simulink model "IEEE30_case"  (R2024b)
settings: Solver=FixedStepAuto  StartTime=0  StopTime=5  FixedStep=1e-7  RelTol=1e-3
values from neighbouring files (symbols this model uses):
  GFL_DFIG_7_C_bus = 0.08    [IEEE30_case_parameters.m]
  GFL_DFIG_7_D_mutual = 2.500000e+3    (= 2500)    [IEEE30_case_parameters.m]
  GFL_DFIG_7_f0 = 60    [IEEE30_case_parameters.m]
  GFL_DFIG_7_gPLLi = 3200    [IEEE30_case_parameters.m]
  GFL_DFIG_7_gPLLp = 650    [IEEE30_case_parameters.m]
  GFL_DFIG_7_H_WT = 0.4    [IEEE30_case_parameters.m]
  GFL_DFIG_7_Hg = 0.8    [IEEE30_case_parameters.m]
  GFL_DFIG_7_Igq_ref = 0    [IEEE30_case_parameters.m]
  GFL_DFIG_7_Ird_ref = 704.45696    [IEEE30_case_parameters.m]
  GFL_DFIG_7_KI_V = -300000    [IEEE30_case_parameters.m]
  GFL_DFIG_7_KP_V = -1000    [IEEE30_case_parameters.m]
  GFL_DFIG_7_Ksh = 1.254300e+4    (= 12543)    [IEEE30_case_parameters.m]
  GFL_DFIG_7_Lg = 0.000483    [IEEE30_case_parameters.m]
  GFL_DFIG_7_Lm_pu = 4    [IEEE30_case_parameters.m]
  GFL_DFIG_7_N = 100    [IEEE30_case_parameters.m]
  GFL_DFIG_7_p = 2    [IEEE30_case_parameters.m]
  GFL_DFIG_7_Pitch = 0    [IEEE30_case_parameters.m]
  GFL_DFIG_7_R = 44    [IEEE30_case_parameters.m]
  GFL_DFIG_7_Rg = 2.000000e-5    (= 2e-05)    [IEEE30_case_parameters.m]
  GFL_DFIG_7_rho = 1.225    [IEEE30_case_parameters.m]
  GFL_DFIG_7_rPLLi = 4500    [IEEE30_case_parameters.m]
  GFL_DFIG_7_rPLLp = 620    [IEEE30_case_parameters.m]
  GFL_DFIG_7_Rs_pu = 0.011    [IEEE30_case_parameters.m]
  GFL_DFIG_7_Sbase = 2.000000e+6    (= 2000000)    [IEEE30_case_parameters.m]
  GFL_DFIG_7_ugq_ref = 0    [IEEE30_case_parameters.m]
  GFL_DFIG_7_usd_ref = 0    [IEEE30_case_parameters.m]
  GFL_DFIG_7_Vbase = 690    [IEEE30_case_parameters.m]
  GFL_DFIG_7_Vdc_ref = 1200    [IEEE30_case_parameters.m]
  GFL_DFIG_7_wind = 12    [IEEE30_case_parameters.m]
  GFL_DFIG_7_wm_ref = 518.184209    [IEEE30_case_parameters.m]
  SG_D_13_D = 0.01056    [IEEE30_case_parameters.m]
  SG_D_13_EnableSaturation = 0    [IEEE30_case_parameters.m]
  SG_D_13_f0 = 60    [IEEE30_case_parameters.m]
  SG_D_13_H = 7.5    [IEEE30_case_parameters.m]
  SG_D_13_K_A = 20    [IEEE30_case_parameters.m]
  SG_D_13_K_E = 1.000000e+1    (= 10)    [IEEE30_case_parameters.m]
  SG_D_13_K_F = 2.363    [IEEE30_case_parameters.m]
  SG_D_13_K_s = 0.5    [IEEE30_case_parameters.m]
  SG_D_13_R_a = 0.001088    [IEEE30_case_parameters.m]
  SG_D_13_S_A = 1    [IEEE30_case_parameters.m]
  SG_D_13_S_B = 0.103    [IEEE30_case_parameters.m]
  SG_D_13_S_N = 10.659857    [IEEE30_case_parameters.m]
  SG_D_13_SpeedPara = 200    [IEEE30_case_parameters.m]
  SG_D_13_T_0 = 0.370163    [IEEE30_case_parameters.m]
  SG_D_13_T_1 = 0.3    [IEEE30_case_parameters.m]
  SG_D_13_T_2 = 0.05    [IEEE30_case_parameters.m]
  SG_D_13_T_3 = 0.02    [IEEE30_case_parameters.m]
  SG_D_13_T_4 = 0.005    [IEEE30_case_parameters.m]
  SG_D_13_T_A = 0.02    [IEEE30_case_parameters.m]
  SG_D_13_T_dd = 8.000000e+0    (= 8)    [IEEE30_case_parameters.m]
  SG_D_13_T_ddd = 0.04    [IEEE30_case_parameters.m]
  SG_D_13_T_E = 0.314    [IEEE30_case_parameters.m]
  SG_D_13_T_F = 0.35    [IEEE30_case_parameters.m]
  SG_D_13_T_qd = 0.8    [IEEE30_case_parameters.m]
  SG_D_13_T_qdd = 0.02    [IEEE30_case_parameters.m]
  SG_D_13_T_speed = 0.1    [IEEE30_case_parameters.m]
  SG_D_13_T_w = 0.5    [IEEE30_case_parameters.m]
  SG_D_13_V_ref = 1.696619    [IEEE30_case_parameters.m]
  SG_D_13_w_ref = 376.991118    [IEEE30_case_parameters.m]
  SG_D_13_x_d = 1.9    [IEEE30_case_parameters.m]
  SG_D_13_x_dd = 0.302    [IEEE30_case_parameters.m]
  SG_D_13_x_ddd = 0.204    [IEEE30_case_parameters.m]
  SG_D_13_x_l = 0.05    [IEEE30_case_parameters.m]
  SG_D_13_x_q = 1.3    [IEEE30_case_parameters.m]
  SG_D_13_x_qd = 0.5    [IEEE30_case_parameters.m]
  SG_D_13_x_qdd = 0.3    [IEEE30_case_parameters.m]
  SG_D_1_D = 0.01056    [IEEE30_case_parameters.m]
  SG_D_1_EnableSaturation = 0    [IEEE30_case_parameters.m]
  SG_D_1_f0 = 60    [IEEE30_case_parameters.m]
  SG_D_1_H = 7.5    [IEEE30_case_parameters.m]
  SG_D_1_K_A = 20    [IEEE30_case_parameters.m]
  SG_D_1_K_E = 1.000000e+1    (= 10)    [IEEE30_case_parameters.m]
  SG_D_1_K_F = 2.363    [IEEE30_case_parameters.m]
  SG_D_1_K_s = 0.5    [IEEE30_case_parameters.m]
  SG_D_1_R_a = 0.001088    [IEEE30_case_parameters.m]
  SG_D_1_S_A = 1    [IEEE30_case_parameters.m]
  SG_D_1_S_B = 0.103    [IEEE30_case_parameters.m]
  SG_D_1_S_N = 10.659857    [IEEE30_case_parameters.m]
  SG_D_1_SpeedPara = 200    [IEEE30_case_parameters.m]
  SG_D_1_T_0 = 0.259812    [IEEE30_case_parameters.m]
  SG_D_1_T_1 = 0.3    [IEEE30_case_parameters.m]
  SG_D_1_T_2 = 0.05    [IEEE30_case_parameters.m]
  SG_D_1_T_3 = 0.02    [IEEE30_case_parameters.m]
  SG_D_1_T_4 = 0.005    [IEEE30_case_parameters.m]
  SG_D_1_T_A = 0.02    [IEEE30_case_parameters.m]
  SG_D_1_T_dd = 8.000000e+0    (= 8)    [IEEE30_case_parameters.m]
  SG_D_1_T_ddd = 0.04    [IEEE30_case_parameters.m]
  SG_D_1_T_E = 0.314    [IEEE30_case_parameters.m]
  SG_D_1_T_F = 0.35    [IEEE30_case_parameters.m]
  SG_D_1_T_qd = 0.8    [IEEE30_case_parameters.m]
  SG_D_1_T_qdd = 0.02    [IEEE30_case_parameters.m]
  SG_D_1_T_speed = 0.1    [IEEE30_case_parameters.m]
  SG_D_1_T_w = 0.5    [IEEE30_case_parameters.m]
  SG_D_1_V_ref = 1.544107    [IEEE30_case_parameters.m]
  SG_D_1_w_ref = 376.991118    [IEEE30_case_parameters.m]
  SG_D_1_x_d = 1.9    [IEEE30_case_parameters.m]
  SG_D_1_x_dd = 0.302    [IEEE30_case_parameters.m]
  SG_D_1_x_ddd = 0.204    [IEEE30_case_parameters.m]
  SG_D_1_x_l = 0.05    [IEEE30_case_parameters.m]
  SG_D_1_x_q = 1.3    [IEEE30_case_parameters.m]
  SG_D_1_x_qd = 0.5    [IEEE30_case_parameters.m]
  SG_D_1_x_qdd = 0.3    [IEEE30_case_parameters.m]
  SG_D_22_D = 0.01056    [IEEE30_case_parameters.m]
  SG_D_22_EnableSaturation = 0    [IEEE30_case_parameters.m]
  SG_D_22_f0 = 60    [IEEE30_case_parameters.m]
  SG_D_22_H = 7.5    [IEEE30_case_parameters.m]
  SG_D_22_K_A = 20    [IEEE30_case_parameters.m]
  SG_D_22_K_E = 1.000000e+1    (= 10)    [IEEE30_case_parameters.m]
  SG_D_22_K_F = 2.363    [IEEE30_case_parameters.m]
  SG_D_22_K_s = 0.5    [IEEE30_case_parameters.m]
  SG_D_22_R_a = 0.001088    [IEEE30_case_parameters.m]
  SG_D_22_S_A = 1    [IEEE30_case_parameters.m]
  SG_D_22_S_B = 0.103    [IEEE30_case_parameters.m]
  SG_D_22_S_N = 10.659857    [IEEE30_case_parameters.m]
  SG_D_22_SpeedPara = 200    [IEEE30_case_parameters.m]
  SG_D_22_T_0 = 0.216121    [IEEE30_case_parameters.m]
  SG_D_22_T_1 = 0.3    [IEEE30_case_parameters.m]
  SG_D_22_T_2 = 0.05    [IEEE30_case_parameters.m]
  SG_D_22_T_3 = 0.02    [IEEE30_case_parameters.m]
  SG_D_22_T_4 = 0.005    [IEEE30_case_parameters.m]
  ... (+126 more)
(part 16 of 27)

== system IEEE30_case/SG_D_1/d_Px_2_SG_D_1_block ==
  note: d_Px_2_SG_D_1 in IEEE30_case
      | $\frac{\mathrm{Px}_{1,\mathrm{SG},D,1}-T_{2}\,\left(\frac{\mathrm{Px}_{1,\mathrm{SG},D,1}}{T_{w}}-\frac{w_{\mathrm{SG},D,1}-2\,\pi \,f_{0}}{T_{w}}\right)}{T_{1}}-\frac{\mathrm{Px}_{2,\mathrm{SG},D,1}}{T_{1}}$
      | Automatically generated on 2025-11-01 18:30:40 .
  State_Px_2_SG_D_1_7ad78 : Inport
  State_Px_1_SG_D_1_ae78a : Inport  Port=2
  State_Px_1_SG_D_1_3856c : Inport  Port=3
  State_w_SG_D_1_34181 : Inport  Port=4
  Add_14e72 : Sum
  Add_312b6 : Sum
  Add_4af92 : Sum
  Add_c84e5 : Sum
  Constant_-1_0a70e : Constant  Value=-1
  Constant_-1_b2e32 : Constant  Value=-1
  Constant_-2.0_99803 : Constant  Value=-2.0
  Constant_T_1_53d02 : Constant  Value=T_1
  Constant_T_1_b414e : Constant  Value=T_1
  Constant_T_2_fd2a1 : Constant  Value=T_2
  Constant_T_w_8633f : Constant  Value=T_w
  Constant_T_w_a9709 : Constant  Value=T_w
  Constant_f0_f4a44 : Constant  Value=f0
  Constant_pi_968ef : Constant  Value=pi
  Divide_043e7 : Product  Inputs=*/
  Divide_4ff0b : Product  Inputs=*/
  Divide_5a47e : Product  Inputs=*/
  Divide_e1124 : Product  Inputs=*/
  Product_026fd : Product
  Product_1f51f : Product
  Product_38c4f : Product
  Product_a5094 : Product
  Product_e3861 : Product
  Blockout_d_Px_2_SG_D_1_8ee22 : Outport
  wires:
  Constant_-2.0_99803/1 -> Product_1f51f/1
  State_w_SG_D_1_34181/1 -> Add_14e72/2
  Constant_f0_f4a44/1 -> Product_38c4f/2
  Constant_pi_968ef/1 -> Product_1f51f/2
  Add_c84e5/1 -> Product_026fd/2
  Product_38c4f/1 -> Add_14e72/1
  Divide_5a47e/1 -> Add_c84e5/1
  Product_1f51f/1 -> Product_38c4f/1
  Constant_T_w_8633f/1 -> Divide_5a47e/2
  Constant_-1_b2e32/1 -> Product_e3861/1
  State_Px_1_SG_D_1_3856c/1 -> Product_e3861/2
  Divide_e1124/1 -> Add_312b6/1
  Product_e3861/1 -> Divide_5a47e/1
  Add_14e72/1 -> Divide_4ff0b/1
  Constant_T_w_a9709/1 -> Divide_4ff0b/2
  Divide_4ff0b/1 -> Add_c84e5/2
  Constant_T_2_fd2a1/1 -> Product_026fd/1
  Constant_-1_0a70e/1 -> Product_a5094/1
  State_Px_2_SG_D_1_7ad78/1 -> Product_a5094/2
  State_Px_1_SG_D_1_ae78a/1 -> Add_4af92/1
  Product_026fd/1 -> Add_4af92/2
  Add_4af92/1 -> Divide_043e7/1
  Product_a5094/1 -> Divide_e1124/1
  Constant_T_1_b414e/1 -> Divide_e1124/2
  Constant_T_1_53d02/1 -> Divide_043e7/2
  Divide_043e7/1 -> Add_312b6/2
  Add_312b6/1 -> Blockout_d_Px_2_SG_D_1_8ee22/1

== system IEEE30_case/SG_D_1/d_Px_3_SG_D_1_block ==
  note: d_Px_3_SG_D_1 in IEEE30_case
      | $\frac{\mathrm{Px}_{2,\mathrm{SG},D,1}+T_{4}\,\left(\frac{\mathrm{Px}_{1,\mathrm{SG},D,1}-T_{2}\,\left(\frac{\mathrm{Px}_{1,\mathrm{SG},D,1}}{T_{w}}-\frac{w_{\mathrm{SG},D,1}-2\,\pi \,f_{0}}{T_{w}}\right)}{T_{1}}-\frac{\mathrm{Px}_{2,\mathrm{SG},D,1}}{T_{1}}\right)}{T_{3}}-\frac{\mathrm{Px}_{3,\mathrm{SG},D,1}}{T_{3}}$
      | Automatically generated on 2025-11-01 18:30:42 .
  State_Px_3_SG_D_1_caa78 : Inport
  State_Px_2_SG_D_1_d9b49 : Inport  Port=2
  State_Px_2_SG_D_1_ab48e : Inport  Port=3
  State_Px_1_SG_D_1_64472 : Inport  Port=4
  State_Px_1_SG_D_1_665ee : Inport  Port=5
  State_w_SG_D_1_e8e94 : Inport  Port=6
  Add_09c98 : Sum
  Add_369a2 : Sum
  Add_66d7b : Sum
  Add_a0e61 : Sum
  Add_c7021 : Sum
  Add_fc02d : Sum
  Constant_-1_a8f79 : Constant  Value=-1
  Constant_-1_ad1eb : Constant  Value=-1
  Constant_-1_fba85 : Constant  Value=-1
  Constant_-2.0_11787 : Constant  Value=-2.0
  Constant_T_1_05b56 : Constant  Value=T_1
  Constant_T_1_e9ffc : Constant  Value=T_1
  Constant_T_2_5461d : Constant  Value=T_2
  Constant_T_3_767c3 : Constant  Value=T_3
  Constant_T_3_e091a : Constant  Value=T_3
  Constant_T_4_12645 : Constant  Value=T_4
  Constant_T_w_0ee7d : Constant  Value=T_w
  Constant_T_w_88f0f : Constant  Value=T_w
  Constant_f0_a696c : Constant  Value=f0
  Constant_pi_8c04d : Constant  Value=pi
  Divide_5430c : Product  Inputs=*/
  Divide_8ac43 : Product  Inputs=*/
  Divide_bb2bd : Product  Inputs=*/
  Divide_c4060 : Product  Inputs=*/
  Divide_c4299 : Product  Inputs=*/
  Divide_d25e4 : Product  Inputs=*/
  Product_246d8 : Product
  Product_55427 : Product
  Product_581c9 : Product
  Product_5bfea : Product
  Product_96dfd : Product
  Product_c40fa : Product
  Product_cae64 : Product
  Blockout_d_Px_3_SG_D_1_3bf99 : Outport
  wires:
  Constant_T_w_88f0f/1 -> Divide_c4299/2
  Constant_-1_ad1eb/1 -> Product_96dfd/1
  Add_fc02d/1 -> Blockout_d_Px_3_SG_D_1_3bf99/1
  Constant_-2.0_11787/1 -> Product_581c9/1
  State_w_SG_D_1_e8e94/1 -> Add_369a2/2
  Constant_f0_a696c/1 -> Product_cae64/2
  State_Px_1_SG_D_1_665ee/1 -> Product_96dfd/2
  Constant_pi_8c04d/1 -> Product_581c9/2
  Product_cae64/1 -> Add_369a2/1
  Product_581c9/1 -> Product_cae64/1
  Product_96dfd/1 -> Divide_c4299/1
  Divide_bb2bd/1 -> Add_fc02d/1
  Constant_T_3_e091a/1 -> Divide_8ac43/2
  Add_369a2/1 -> Divide_d25e4/1
  Constant_T_w_0ee7d/1 -> Divide_d25e4/2
  Divide_c4299/1 -> Add_a0e61/1
  Divide_d25e4/1 -> Add_a0e61/2
  Constant_-1_fba85/1 -> Product_246d8/1
  Constant_T_2_5461d/1 -> Product_c40fa/1
  Add_a0e61/1 -> Product_c40fa/2
  Constant_-1_a8f79/1 -> Product_5bfea/1
  Divide_8ac43/1 -> Add_fc02d/2
  Constant_T_3_767c3/1 -> Divide_bb2bd/2
  State_Px_2_SG_D_1_ab48e/1 -> Product_5bfea/2
  State_Px_1_SG_D_1_64472/1 -> Add_66d7b/1
  Divide_c4060/1 -> Add_c7021/1
  Product_c40fa/1 -> Add_66d7b/2
  Product_5bfea/1 -> Divide_c4060/1
  Product_246d8/1 -> Divide_bb2bd/1
  Constant_T_1_05b56/1 -> Divide_c4060/2
  Add_66d7b/1 -> Divide_5430c/1
  Constant_T_1_e9ffc/1 -> Divide_5430c/2
  Divide_5430c/1 -> Add_c7021/2
  Constant_T_4_12645/1 -> Product_55427/1
  Add_c7021/1 -> Product_55427/2
  State_Px_3_SG_D_1_caa78/1 -> Product_246d8/2
  State_Px_2_SG_D_1_d9b49/1 -> Add_09c98/1
  Product_55427/1 -> Add_09c98/2
  Add_09c98/1 -> Divide_8ac43/1

== system IEEE30_case/SG_D_1/d_R_f_SG_D_1_block ==
  note: d_R_f_SG_D_1 in IEEE30_case
      | $-\frac{R_{f,\mathrm{SG},D,1}-\frac{E_{\mathrm{fd},\mathrm{SG},D,1}\,K_{F}}{T_{F}}}{T_{F}}$
      | Automatically generated on 2025-11-01 18:30:36 .
  State_E_fd_SG_D_1_7bfd0 : Inport
  State_R_f_SG_D_1_11fa9 : Inport  Port=2
  Constant_K_F_288dd : Constant  Value=K_F
  Constant_T_F_528c7 : Constant  Value=T_F
  Constant_T_F_87a06 : Constant  Value=T_F
  Divide_3eb50 : Product  Inputs=*/
  Divide_9ebff : Product  Inputs=*/
  Product_09a34 : Product
  Subtract_13a9b : Sum  Inputs=+-
  Blockout_d_R_f_SG_D_1_cb206 : Outport
  wires:
  Constant_K_F_288dd/1 -> Product_09a34/2
  Product_09a34/1 -> Divide_3eb50/1
  State_E_fd_SG_D_1_7bfd0/1 -> Product_09a34/1
  State_R_f_SG_D_1_11fa9/1 -> Subtract_13a9b/2
  Constant_T_F_528c7/1 -> Divide_3eb50/2
  Divide_3eb50/1 -> Subtract_13a9b/1
  Divide_9ebff/1 -> Blockout_d_R_f_SG_D_1_cb206/1
  Subtract_13a9b/1 -> Divide_9ebff/1
  Constant_T_F_87a06/1 -> Divide_9ebff/2

== system IEEE30_case/SG_D_1/d_T_m_SG_D_1_block ==
  note: d_T_m_SG_D_1 in IEEE30_case
      | $-\frac{T_{m,\mathrm{SG},D,1}-T_{0}+\frac{\mathrm{SpeedPara}\,\left(w_{\mathrm{SG},D,1}-w_{\mathrm{ref}}\right)}{2\,f_{0}\,\pi }}{T_{\mathrm{speed}}}$
      | Automatically generated on 2025-11-01 18:30:26 .
  State_w_SG_D_1_e56b0 : Inport
  State_T_m_SG_D_1_eb6d8 : Inport  Port=2
  Add_2376c : Sum
  Add_d3f82 : Sum
  Constant_-1_17636 : Constant  Value=-1
  Constant_2.0_24c8d : Constant  Value=2.0
  Constant_SpeedPara_8f4c6 : Constant  Value=SpeedPara
  Constant_T_0_1fdba : Constant  Value=T_0
  Constant_T_speed_8d11c : Constant  Value=T_speed
  Constant_f0_adcf2 : Constant  Value=f0
  Constant_pi_83027 : Constant  Value=pi
  Constant_w_ref_bad2c : Constant  Value=w_ref
  Divide_03ba9 : Product  Inputs=*/
  Divide_931b1 : Product  Inputs=*/
  Product_038ba : Product
  Product_39944 : Product
  Product_c8531 : Product
  Product_eec2d : Product
  Subtract_6dd9b : Sum  Inputs=+-
  Blockout_d_T_m_SG_D_1_12514 : Outport
  wires:
  Constant_-1_17636/1 -> Product_39944/1
  Constant_w_ref_bad2c/1 -> Add_d3f82/2
  State_w_SG_D_1_e56b0/1 -> Product_39944/2
  Add_2376c/1 -> Subtract_6dd9b/1
  Add_d3f82/1 -> Product_038ba/2
  Product_39944/1 -> Add_d3f82/1
  Constant_2.0_24c8d/1 -> Product_eec2d/1
  Constant_pi_83027/1 -> Product_eec2d/2
  Constant_SpeedPara_8f4c6/1 -> Product_038ba/1
  Product_eec2d/1 -> Product_c8531/1
  Constant_f0_adcf2/1 -> Product_c8531/2
  Constant_T_speed_8d11c/1 -> Divide_931b1/2
  Product_038ba/1 -> Divide_03ba9/1
  Product_c8531/1 -> Divide_03ba9/2
  Divide_03ba9/1 -> Add_2376c/1
  Constant_T_0_1fdba/1 -> Add_2376c/2
  State_T_m_SG_D_1_eb6d8/1 -> Subtract_6dd9b/2
  Subtract_6dd9b/1 -> Divide_931b1/1
  Divide_931b1/1 -> Blockout_d_T_m_SG_D_1_12514/1

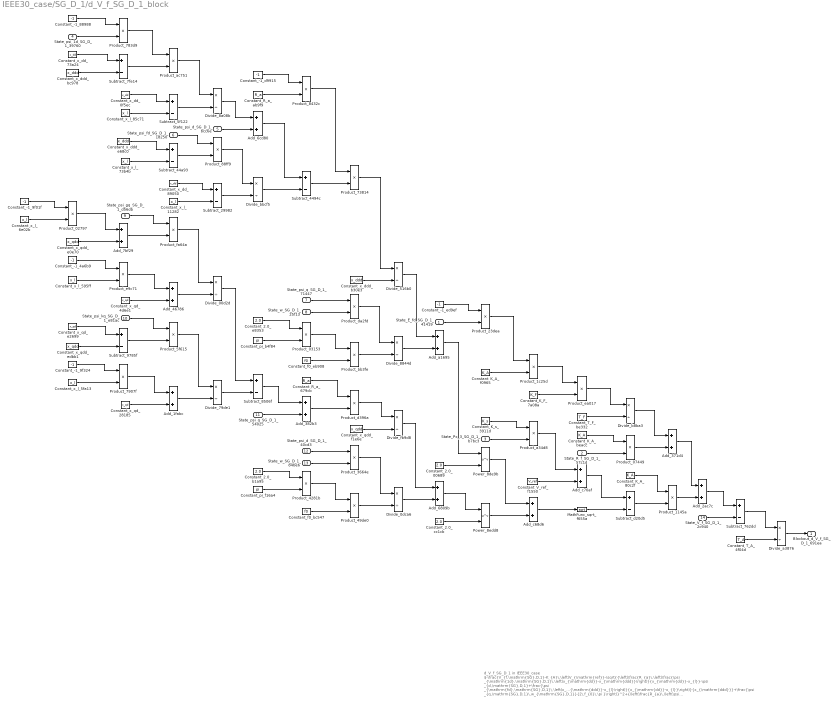
== system IEEE30_case/SG_D_1/d_V_f_SG_D_1_block ==
  note: d_V_f_SG_D_1 in IEEE30_case
      | $-\frac{V_{f,\mathrm{SG},D,1}-K_{A}\,\left(V_{\mathrm{ref}}-\sqrt{{\left(\frac{R_{a}\,\left(\frac{\psi _{\mathrm{1d},\mathrm{SG},D,1}\,\left(x_{\mathrm{dd}}-x_{\mathrm{ddd}}\right)}{x_{\mathrm{dd}}-x_{l}}-\psi _{d,\mathrm{SG},D,1}+\frac{\psi _{\mathrm{fd},\mathrm{SG},D,1}\,\left(x_{\mathrm{ddd}}-x_{l}\right)}{x_{\mathrm{dd}}-x_{l}}\right)}{x_{\mathrm{ddd}}}+\frac{\psi _{q,\mathrm{SG},D,1}\,w_{\mathrm{SG},D,1}}{2\,f_{0}\,\pi }\right)}^2+{\left(\frac{R_{a}\,\left(\psi _{q,\mathrm{SG},D,1}+\frac{\psi _{\mathrm{gq},\mathrm{SG},D,1}\,\left(x_{l}-x_{\mathrm{qdd}}\right)}{x_{l}-x_{\mathrm{qd}}}+\frac{\psi _{\mathrm{kq},\mathrm{SG},D,1}\,\left(x_{\mathrm{qd}}-x_{\mathrm{qdd}}\right)}{x_{l}-x_{\mathrm{qd}}}\right)}{x_{\mathrm{qdd}}}+\frac{\psi _{d,\mathrm{SG},D,1}\,w_{\mathrm{SG},D,1}}{2\,f_{0}\,\pi }\right)}^2}+K_{s}\,\mathrm{Px}_{3,\mathrm{SG},D,1}\right)-K_{A}\,R_{f,\mathrm{SG},D,1}+\frac{E_{\mathrm{fd},\mathrm{SG},D,1}\,K_{A}\,K_{F}}{T_{F}}}{T_{A}}$
      | Automatically generated on 2025-11-01 18:30:34 .
  State_E_fd_SG_D_1_41419 : Inport
  State_R_f_SG_D_1_57c1d : Inport  Port=2
  State_Px_3_SG_D_1_b7bc3 : Inport  Port=3
  State_psi_1d_SG_D_1_39760 : Inport  Port=4
  State_psi_d_SG_D_1_bcc6e : Inport  Port=5
  State_psi_fd_SG_D_1_18250 : Inport  Port=6
  State_psi_q_SG_D_1_71447 : Inport  Port=7
  State_w_SG_D_1_25f13 : Inport  Port=8
  State_psi_gq_SG_D_1_d56db : Inport  Port=9
  State_psi_kq_SG_D_1_e81ac : Inport  Port=10
  State_psi_q_SG_D_1_54025 : Inport  Port=11
  State_psi_d_SG_D_1_40cd3 : Inport  Port=12
  State_w_SG_D_1_84be6 : Inport  Port=13
  State_V_f_SG_D_1_2c940 : Inport  Port=14
  Add_1fabc : Sum
  Add_2ac7c : Sum
  Add_371d4 : Sum
  Add_382b3 : Sum
  Add_46786 : Sum
  Add_6809b : Sum
  Add_6cd80 : Sum
  Add_7bf29 : Sum
  Add_a1695 : Sum
  Add_c68d6 : Sum
  Add_c70af : Sum
  Constant_-1_4a6b9 : Constant  Value=-1
  Constant_-1_88988 : Constant  Value=-1
  Constant_-1_9f01f : Constant  Value=-1
  Constant_-1_9f324 : Constant  Value=-1
  Constant_-1_d9915 : Constant  Value=-1
  Constant_-1_ed9ef : Constant  Value=-1
  Constant_2.0_00689 : Constant  Value=2.0
  Constant_2.0_b1a95 : Constant  Value=2.0
  Constant_2.0_cc1cb : Constant  Value=2.0
  Constant_2.0_e8353 : Constant  Value=2.0
  Constant_K_A_80c2f : Constant  Value=K_A
  Constant_K_A_beacc : Constant  Value=K_A
  Constant_K_A_f0965 : Constant  Value=K_A
  Constant_K_F_7a08a : Constant  Value=K_F
  Constant_K_s_3911d : Constant  Value=K_s
  Constant_R_a_679cb : Constant  Value=R_a
  Constant_R_a_ab9f9 : Constant  Value=R_a
  Constant_T_A_4f04d : Constant  Value=T_A
  Constant_T_F_be332 : Constant  Value=T_F
  Constant_V_ref_f1550 : Constant  Value=V_ref
  Constant_f0_bc547 : Constant  Value=f0
  Constant_f0_eb908 : Constant  Value=f0
  Constant_pi_b4f84 : Constant  Value=pi
  Constant_pi_f16a4 : Constant  Value=pi
  Constant_x_dd_0f5ec : Constant  Value=x_dd
  Constant_x_dd_73a24 : Constant  Value=x_dd
  Constant_x_dd_89050 : Constant  Value=x_dd
  Constant_x_ddd_b30e3 : Constant  Value=x_ddd
  Constant_x_ddd_bc978 : Constant  Value=x_ddd
  Constant_x_ddd_e68c0 : Constant  Value=x_ddd
  Constant_x_l_11282 : Constant  Value=x_l
  Constant_x_l_595ff : Constant  Value=x_l
  Constant_x_l_5fa13 : Constant  Value=x_l
  Constant_x_l_6e02b : Constant  Value=x_l
  Constant_x_l_73b4b : Constant  Value=x_l
  Constant_x_l_85c71 : Constant  Value=x_l
  Constant_x_qd_28185 : Constant  Value=x_qd
  Constant_x_qd_4d6e1 : Constant  Value=x_qd
  Constant_x_qd_e2699 : Constant  Value=x_qd
  Constant_x_qdd_e0e70 : Constant  Value=x_qdd
  Constant_x_qdd_edbb1 : Constant  Value=x_qdd
  Constant_x_qdd_f1e6e : Constant  Value=x_qdd
  Divide_00d2d : Product  Inputs=*/
  Divide_0dca6 : Product  Inputs=*/
  Divide_516b0 : Product  Inputs=*/
  Divide_79de1 : Product  Inputs=*/
  Divide_8844d : Product  Inputs=*/
  Divide_8a08b : Product  Inputs=*/
  Divide_a3876 : Product  Inputs=*/
  Divide_b8ba3 : Product  Inputs=*/
  Divide_bbcf5 : Product  Inputs=*/
  Divide_fb9d8 : Product  Inputs=*/
  MathFunc_sqrt_f655a : Sqrt
  Power_8de9b : Math  Operator=pow
  Power_8edd8 : Math  Operator=pow
  Product_02797 : Product
  Product_03153 : Product
  Product_07449 : Product
  Product_1145a : Product
  Product_1c25d : Product
  Product_23dea : Product
  Product_3664e : Product
  Product_4281b : Product
  Product_49de0 : Product
  Product_5f615 : Product
  Product_73814 : Product
  Product_783d9 : Product
  Product_7907f : Product
  Product_8432c : Product
  Product_88ff9 : Product
  Product_a34d8 : Product
  Product_ac751 : Product
  Product_bb3fe : Product
  Product_d396a : Product
  Product_da2fd : Product
  Product_e9c71 : Product
  Product_ea017 : Product
  Product_fa64a : Product
  Subtract_29982 : Sum  Inputs=+-
  Subtract_4494c : Sum  Inputs=+-
  Subtract_44a93 : Sum  Inputs=+-
  Subtract_5f122 : Sum  Inputs=+-
  Subtract_762dd : Sum  Inputs=+-
  Subtract_7fe14 : Sum  Inputs=+-
  Subtract_8506f : Sum  Inputs=+-
  Subtract_9785f : Sum  Inputs=+-
  Subtract_d20d5 : Sum  Inputs=+-
  Blockout_d_V_f_SG_D_1_691ea : Outport
  wires:
  Constant_-1_9f324/1 -> Product_7907f/1
  Constant_-1_9f01f/1 -> Product_02797/1
  State_psi_d_SG_D_1_40cd3/1 -> Product_3664e/1
  Constant_x_qd_28185/1 -> Add_1fabc/2
  Constant_x_qdd_e0e70/1 -> Add_7bf29/2
  State_w_SG_D_1_84be6/1 -> Product_3664e/2
  Constant_x_l_6e02b/1 -> Product_02797/2
  Subtract_4494c/1 -> Product_73814/2
  Constant_x_l_5fa13/1 -> Product_7907f/2
  Constant_x_dd_73a24/1 -> Subtract_7fe14/1
  Constant_R_a_ab9f9/1 -> Product_8432c/2
  Constant_-1_88988/1 -> Product_783d9/1
  Divide_bbcf5/1 -> Subtract_4494c/2
  Constant_x_ddd_bc978/1 -> Subtract_7fe14/2
  Add_1fabc/1 -> Divide_79de1/2
  State_psi_1d_SG_D_1_39760/1 -> Product_783d9/2
  Add_46786/1 -> Divide_00d2d/2
  Subtract_9785f/1 -> Product_5f615/2
  Product_ea017/1 -> Divide_b8ba3/1
  Product_03153/1 -> Product_bb3fe/1
  Product_02797/1 -> Add_7bf29/1
  Constant_-1_4a6b9/1 -> Product_e9c71/1
  Constant_x_l_595ff/1 -> Product_e9c71/2
  Add_6cd80/1 -> Subtract_4494c/1
  Constant_2.0_b1a95/1 -> Product_4281b/1
  Constant_x_qd_e2699/1 -> Subtract_9785f/1
  Product_783d9/1 -> Product_ac751/1
  Constant_pi_f16a4/1 -> Product_4281b/2
  Constant_x_qdd_edbb1/1 -> Subtract_9785f/2
  Subtract_7fe14/1 -> Product_ac751/2
  State_psi_q_SG_D_1_54025/1 -> Add_382b3/2
  Constant_x_dd_0f5ec/1 -> Subtract_5f122/1
  Constant_x_l_85c71/1 -> Subtract_5f122/2
  Constant_x_ddd_e68c0/1 -> Subtract_44a93/1
  Constant_x_l_73b4b/1 -> Subtract_44a93/2
  State_psi_gq_SG_D_1_d56db/1 -> Product_fa64a/1
  Add_7bf29/1 -> Product_fa64a/2
  Product_e9c71/1 -> Add_46786/1
  Constant_x_qd_4d6e1/1 -> Add_46786/2
  Divide_8a08b/1 -> Add_6cd80/1
  Subtract_5f122/1 -> Divide_8a08b/2
  State_psi_kq_SG_D_1_e81ac/1 -> Product_5f615/1
  Divide_a3876/1 -> Blockout_d_V_f_SG_D_1_691ea/1
  Product_7907f/1 -> Add_1fabc/1
  Product_ac751/1 -> Divide_8a08b/1
  State_psi_fd_SG_D_1_18250/1 -> Product_88ff9/1
  State_w_SG_D_1_25f13/1 -> Product_da2fd/2
  Subtract_44a93/1 -> Product_88ff9/2
  Constant_x_dd_89050/1 -> Subtract_29982/1
  Constant_x_l_11282/1 -> Subtract_29982/2
  Product_fa64a/1 -> Divide_00d2d/1
  Product_8432c/1 -> Product_73814/1
  Product_5f615/1 -> Divide_79de1/1
  State_psi_d_SG_D_1_bcc6e/1 -> Add_6cd80/2
  Product_88ff9/1 -> Divide_bbcf5/1
  Subtract_29982/1 -> Divide_bbcf5/2
  Divide_00d2d/1 -> Subtract_8506f/1
  Divide_79de1/1 -> Subtract_8506f/2
  Constant_-1_d9915/1 -> Product_8432c/1
  Constant_2.0_e8353/1 -> Product_03153/1
  Constant_pi_b4f84/1 -> Product_03153/2
  Subtract_8506f/1 -> Add_382b3/1
  State_psi_q_SG_D_1_71447/1 -> Product_da2fd/1
  Constant_f0_eb908/1 -> Product_bb3fe/2
  Constant_R_a_679cb/1 -> Product_d396a/1
  Add_382b3/1 -> Product_d396a/2
  Product_4281b/1 -> Product_49de0/1
  Power_8de9b/1 -> Add_c68d6/1
  Constant_f0_bc547/1 -> Product_49de0/2
  Product_73814/1 -> Divide_516b0/1
  Constant_x_ddd_b30e3/1 -> Divide_516b0/2
  Product_da2fd/1 -> Divide_8844d/1
  Product_bb3fe/1 -> Divide_8844d/2
  Product_d396a/1 -> Divide_fb9d8/1
  Constant_x_qdd_f1e6e/1 -> Divide_fb9d8/2
  Product_3664e/1 -> Divide_0dca6/1
  Product_49de0/1 -> Divide_0dca6/2
  Divide_516b0/1 -> Add_a1695/1
  Divide_8844d/1 -> Add_a1695/2
  Divide_fb9d8/1 -> Add_6809b/1
  Divide_0dca6/1 -> Add_6809b/2
  Constant_-1_ed9ef/1 -> Product_23dea/1
  State_E_fd_SG_D_1_41419/1 -> Product_23dea/2
  Add_a1695/1 -> Power_8de9b/1
  Constant_2.0_00689/1 -> Power_8de9b/2
  Add_6809b/1 -> Power_8edd8/1
  Constant_2.0_cc1cb/1 -> Power_8edd8/2
  Product_23dea/1 -> Product_1c25d/1
  Constant_K_A_f0965/1 -> Product_1c25d/2
  Constant_K_s_3911d/1 -> Product_a34d8/1
  State_Px_3_SG_D_1_b7bc3/1 -> Product_a34d8/2
  Power_8edd8/1 -> Add_c68d6/2
  Divide_b8ba3/1 -> Add_371d4/1
  Product_1c25d/1 -> Product_ea017/1
  Constant_K_F_7a08a/1 -> Product_ea017/2
  Product_a34d8/1 -> Add_c70af/1
  Constant_V_ref_f1550/1 -> Add_c70af/2
  Add_c68d6/1 -> MathFunc_sqrt_f655a/1
  Constant_T_F_be332/1 -> Divide_b8ba3/2
  Constant_K_A_beacc/1 -> Product_07449/1
  State_R_f_SG_D_1_57c1d/1 -> Product_07449/2
  Add_c70af/1 -> Subtract_d20d5/1
  MathFunc_sqrt_f655a/1 -> Subtract_d20d5/2
  Constant_T_A_4f04d/1 -> Divide_a3876/2
  Product_07449/1 -> Add_371d4/2
  Constant_K_A_80c2f/1 -> Product_1145a/1
  Subtract_d20d5/1 -> Product_1145a/2
  Add_371d4/1 -> Add_2ac7c/1
  Product_1145a/1 -> Add_2ac7c/2
  Add_2ac7c/1 -> Subtract_762dd/1
  State_V_f_SG_D_1_2c940/1 -> Subtract_762dd/2
  Subtract_762dd/1 -> Divide_a3876/1

== system IEEE30_case/SG_D_1/d_psi_1d_SG_D_1_block ==
  note: d_psi_1d_SG_D_1 in IEEE30_case
      | $-\frac{\psi _{\mathrm{1d},\mathrm{SG},D,1}-\psi _{\mathrm{fd},\mathrm{SG},D,1}+\frac{\left(x_{\mathrm{dd}}-x_{l}\right)\,\left(\frac{\psi _{\mathrm{1d},\mathrm{SG},D,1}\,\left(x_{\mathrm{dd}}-x_{\mathrm{ddd}}\right)}{x_{\mathrm{dd}}-x_{l}}-\psi _{d,\mathrm{SG},D,1}+\frac{\psi _{\mathrm{fd},\mathrm{SG},D,1}\,\left(x_{\mathrm{ddd}}-x_{l}\right)}{x_{\mathrm{dd}}-x_{l}}\right)}{x_{\mathrm{ddd}}}}{T_{\mathrm{ddd}}}$
      | Automatically generated on 2025-11-01 18:30:08 .
  State_psi_1d_SG_D_1_acde6 : Inport
  State_psi_fd_SG_D_1_697dc : Inport  Port=2
  State_psi_1d_SG_D_1_d153a : Inport  Port=3
  State_psi_d_SG_D_1_ee12b : Inport  Port=4
  State_psi_fd_SG_D_1_a7ee9 : Inport  Port=5
  Add_5282d : Sum
  Add_52e71 : Sum
  Add_8db4e : Sum
  Constant_-1_12fb9 : Constant  Value=-1
  Constant_-1_da2b3 : Constant  Value=-1
  Constant_T_ddd_a3ac7 : Constant  Value=T_ddd
  Constant_x_dd_811ab : Constant  Value=x_dd
  Constant_x_dd_9202a : Constant  Value=x_dd
  Constant_x_dd_93c5d : Constant  Value=x_dd
  Constant_x_dd_b2d25 : Constant  Value=x_dd
  Constant_x_ddd_22811 : Constant  Value=x_ddd
  Constant_x_ddd_71fa5 : Constant  Value=x_ddd
  Constant_x_ddd_90b96 : Constant  Value=x_ddd
  Constant_x_l_1248a : Constant  Value=x_l
  Constant_x_l_4abbc : Constant  Value=x_l
  Constant_x_l_52946 : Constant  Value=x_l
  Constant_x_l_85f89 : Constant  Value=x_l
  Divide_024ae : Product  Inputs=*/
  Divide_23a68 : Product  Inputs=*/
  Divide_6eb96 : Product  Inputs=*/
  Divide_acb20 : Product  Inputs=*/
  Product_30929 : Product
  Product_739fc : Product
  Product_9bbd6 : Product
  Product_d4260 : Product
  Product_d919b : Product
  Subtract_21dd2 : Sum  Inputs=+-
  Subtract_3d153 : Sum  Inputs=+-
  Subtract_7c245 : Sum  Inputs=+-
  Subtract_8b3b8 : Sum  Inputs=+-
  Subtract_9628b : Sum  Inputs=+-
  Subtract_e1559 : Sum  Inputs=+-
  Blockout_d_psi_1d_SG_D_1_c059e : Outport
  wires:
  Product_d919b/1 -> Product_9bbd6/1
  Constant_-1_12fb9/1 -> Product_d919b/1
  Subtract_7c245/1 -> Product_9bbd6/2
  State_psi_1d_SG_D_1_d153a/1 -> Product_d919b/2
  Subtract_9628b/1 -> Product_30929/1
  State_psi_d_SG_D_1_ee12b/1 -> Add_52e71/2
  Constant_x_dd_b2d25/1 -> Subtract_8b3b8/1
  Constant_x_l_85f89/1 -> Subtract_9628b/2
  Constant_x_dd_811ab/1 -> Subtract_7c245/1
  Subtract_3d153/1 -> Product_d4260/2
  Constant_x_l_1248a/1 -> Subtract_8b3b8/2
  Divide_acb20/1 -> Subtract_21dd2/2
  Constant_x_ddd_90b96/1 -> Subtract_7c245/2
  Constant_x_ddd_71fa5/1 -> Subtract_3d153/1
  Constant_x_l_4abbc/1 -> Subtract_3d153/2
  Add_8db4e/1 -> Add_5282d/1
  Product_9bbd6/1 -> Divide_6eb96/1
  Divide_23a68/1 -> Add_5282d/2
  Subtract_8b3b8/1 -> Divide_6eb96/2
  State_psi_fd_SG_D_1_a7ee9/1 -> Product_d4260/1
  Constant_x_dd_9202a/1 -> Subtract_e1559/1
  Constant_x_l_52946/1 -> Subtract_e1559/2
  Constant_x_ddd_22811/1 -> Divide_23a68/2
  Subtract_21dd2/1 -> Product_30929/2
  Divide_6eb96/1 -> Add_52e71/1
  Product_d4260/1 -> Divide_acb20/1
  Subtract_e1559/1 -> Divide_acb20/2
  Product_30929/1 -> Divide_23a68/1
  Constant_x_dd_93c5d/1 -> Subtract_9628b/1
  Add_52e71/1 -> Subtract_21dd2/1
  Constant_-1_da2b3/1 -> Product_739fc/1
  State_psi_1d_SG_D_1_acde6/1 -> Product_739fc/2
  Product_739fc/1 -> Add_8db4e/1
  State_psi_fd_SG_D_1_697dc/1 -> Add_8db4e/2
  Add_5282d/1 -> Divide_024ae/1
  Constant_T_ddd_a3ac7/1 -> Divide_024ae/2
  Divide_024ae/1 -> Blockout_d_psi_1d_SG_D_1_c059e/1

== system IEEE30_case/SG_D_1/d_psi_d_SG_D_1_block ==
  note: d_psi_d_SG_D_1 in IEEE30_case
      | $2\,\pi \,f_{0}\,\left(v_{d,\mathrm{SG},D,1}\,\sin\left(\theta _{\mathrm{SG},D,1}\right)-v_{q,\mathrm{SG},D,1}\,\cos\left(\theta _{\mathrm{SG},D,1}\right)+\frac{R_{a}\,\left(\frac{\psi _{\mathrm{1d},\mathrm{SG},D,1}\,\left(x_{\mathrm{dd}}-x_{\mathrm{ddd}}\right)}{x_{\mathrm{dd}}-x_{l}}-\psi _{d,\mathrm{SG},D,1}+\frac{\psi _{\mathrm{fd},\mathrm{SG},D,1}\,\left(x_{\mathrm{ddd}}-x_{l}\right)}{x_{\mathrm{dd}}-x_{l}}\right)}{x_{\mathrm{ddd}}}+\frac{\psi _{q,\mathrm{SG},D,1}\,w_{\mathrm{SG},D,1}}{2\,f_{0}\,\pi }\right)$
      | Automatically generated on 2025-11-01 18:29:41 .
  State_psi_1d_SG_D_1_5396e : Inport
  State_psi_d_SG_D_1_d85a6 : Inport  Port=2
  State_psi_fd_SG_D_1_f658e : Inport  Port=3
  Input_v_d_SG_D_1_95be5 : Inport  Port=4
  State_theta_SG_D_1_3e828 : Inport  Port=5
  Input_v_q_SG_D_1_f5767 : Inport  Port=6
  State_theta_SG_D_1_93c49 : Inport  Port=7
  State_psi_q_SG_D_1_efd17 : Inport  Port=8
  State_w_SG_D_1_d2cfd : Inport  Port=9
  Add_b2cc0 : Sum
  Add_ec660 : Sum
  Constant_-1_38384 : Constant  Value=-1
  Constant_-2.0_0cf5a : Constant  Value=-2.0
  Constant_2.0_3349a : Constant  Value=2.0
  Constant_R_a_b96de : Constant  Value=R_a
  Constant_f0_4de23 : Constant  Value=f0
  Constant_f0_53b7b : Constant  Value=f0
  Constant_pi_47aad : Constant  Value=pi
  Constant_pi_fd6f4 : Constant  Value=pi
  Constant_x_dd_45d12 : Constant  Value=x_dd
  Constant_x_dd_8310c : Constant  Value=x_dd
  Constant_x_dd_a5eb8 : Constant  Value=x_dd
  Constant_x_ddd_6a29b : Constant  Value=x_ddd
  Constant_x_ddd_832ed : Constant  Value=x_ddd
  Constant_x_ddd_e6836 : Constant  Value=x_ddd
  Constant_x_l_25dcd : Constant  Value=x_l
  Constant_x_l_5e9da : Constant  Value=x_l
  Constant_x_l_ffce5 : Constant  Value=x_l
  Divide_128e2 : Product  Inputs=*/
  Divide_489db : Product  Inputs=*/
  Divide_a41a9 : Product  Inputs=*/
  Divide_c2f47 : Product  Inputs=*/
  MathFunc_cos_86319 : Trigonometry  Operator=cos
  MathFunc_sin_afe2a : Trigonometry
  Product_21064 : Product
  Product_3c407 : Product
  Product_7a831 : Product
  Product_7ef06 : Product
  Product_8cdae : Product
  Product_8d80b : Product
  Product_932e8 : Product
  Product_ba84c : Product
  Product_c21e8 : Product
  Product_cb69a : Product
  Product_e5f81 : Product
  Product_f731f : Product
  Subtract_4b3ee : Sum  Inputs=+-
  Subtract_5a4a0 : Sum  Inputs=+-
  Subtract_6b146 : Sum  Inputs=+-
  Subtract_84717 : Sum  Inputs=+-
  Subtract_a6f20 : Sum  Inputs=+-
  Subtract_aa1cc : Sum  Inputs=+-
  Subtract_dffd2 : Sum  Inputs=+-
  Blockout_d_psi_d_SG_D_1_2866c : Outport
  wires:
  Add_b2cc0/1 -> Subtract_dffd2/1
  Product_7ef06/1 -> Divide_c2f47/1
  Subtract_aa1cc/1 -> Product_7ef06/2
  Divide_c2f47/1 -> Add_b2cc0/1
  Product_3c407/1 -> Product_7ef06/1
  Constant_x_ddd_e6836/1 -> Subtract_aa1cc/2
  Constant_x_dd_45d12/1 -> Subtract_aa1cc/1
  State_psi_1d_SG_D_1_5396e/1 -> Product_3c407/2
  Constant_-1_38384/1 -> Product_3c407/1
  Product_21064/1 -> Divide_128e2/1
  Constant_x_l_ffce5/1 -> Subtract_84717/2
  State_psi_d_SG_D_1_d85a6/1 -> Add_b2cc0/2
  Constant_x_dd_a5eb8/1 -> Subtract_84717/1
  Constant_x_ddd_832ed/1 -> Subtract_a6f20/1
  Constant_x_l_25dcd/1 -> Subtract_a6f20/2
  Subtract_84717/1 -> Divide_c2f47/2
  State_psi_fd_SG_D_1_f658e/1 -> Product_21064/1
  Constant_x_ddd_6a29b/1 -> Divide_489db/2
  Subtract_a6f20/1 -> Product_21064/2
  Product_932e8/1 -> Subtract_5a4a0/2
  Constant_x_dd_8310c/1 -> Subtract_6b146/1
  Constant_x_l_5e9da/1 -> Subtract_6b146/2
  Subtract_6b146/1 -> Divide_128e2/2
  Divide_128e2/1 -> Subtract_dffd2/2
  Constant_R_a_b96de/1 -> Product_e5f81/1
  Subtract_dffd2/1 -> Product_e5f81/2
  MathFunc_cos_86319/1 -> Product_ba84c/2
  State_theta_SG_D_1_3e828/1 -> MathFunc_sin_afe2a/1
  Divide_489db/1 -> Subtract_5a4a0/1
  Product_e5f81/1 -> Divide_489db/1
  MathFunc_sin_afe2a/1 -> Product_932e8/2
  Input_v_d_SG_D_1_95be5/1 -> Product_932e8/1
  Product_8cdae/1 -> Blockout_d_psi_d_SG_D_1_2866c/1
  Product_f731f/1 -> Product_8cdae/1
  Product_7a831/1 -> Product_f731f/1
  State_theta_SG_D_1_93c49/1 -> MathFunc_cos_86319/1
  Constant_2.0_3349a/1 -> Product_8d80b/1
  Constant_pi_47aad/1 -> Product_8d80b/2
  Input_v_q_SG_D_1_f5767/1 -> Product_ba84c/1
  Constant_f0_53b7b/1 -> Product_f731f/2
  State_psi_q_SG_D_1_efd17/1 -> Product_cb69a/1
  State_w_SG_D_1_d2cfd/1 -> Product_cb69a/2
  Product_8d80b/1 -> Product_c21e8/1
  Constant_pi_fd6f4/1 -> Product_7a831/2
  Constant_f0_4de23/1 -> Product_c21e8/2
  Constant_-2.0_0cf5a/1 -> Product_7a831/1
  Add_ec660/1 -> Subtract_4b3ee/1
  Subtract_5a4a0/1 -> Add_ec660/1
  Product_ba84c/1 -> Add_ec660/2
  Product_cb69a/1 -> Divide_a41a9/1
  Product_c21e8/1 -> Divide_a41a9/2
  Divide_a41a9/1 -> Subtract_4b3ee/2
  Subtract_4b3ee/1 -> Product_8cdae/2

== system IEEE30_case/SG_D_1/d_psi_fd_SG_D_1_block ==
  note: d_psi_fd_SG_D_1 in IEEE30_case
      | $-\frac{\psi _{\mathrm{fd},\mathrm{SG},D,1}-E_{\mathrm{fd},\mathrm{SG},D,1}+\left(x_{d}-x_{\mathrm{dd}}\right)\,\left(\frac{\frac{\psi _{\mathrm{1d},\mathrm{SG},D,1}\,\left(x_{\mathrm{dd}}-x_{\mathrm{ddd}}\right)}{x_{\mathrm{dd}}-x_{l}}-\psi _{d,\mathrm{SG},D,1}+\frac{\psi _{\mathrm{fd},\mathrm{SG},D,1}\,\left(x_{\mathrm{ddd}}-x_{l}\right)}{x_{\mathrm{dd}}-x_{l}}}{x_{\mathrm{ddd}}}-\frac{\left(x_{\mathrm{dd}}-x_{\mathrm{ddd}}\right)\,\left(\psi _{\mathrm{1d},\mathrm{SG},D,1}-\psi _{\mathrm{fd},\mathrm{SG},D,1}+\frac{\left(x_{\mathrm{dd}}-x_{l}\right)\,\left(\frac{\psi _{\mathrm{1d},\mathrm{SG},D,1}\,\left(x_{\mathrm{dd}}-x_{\mathrm{ddd}}\right)}{x_{\mathrm{dd}}-x_{l}}-\psi _{d,\mathrm{SG},D,1}+\frac{\psi _{\mathrm{fd},\mathrm{SG},D,1}\,\left(x_{\mathrm{ddd}}-x_{l}\right)}{x_{\mathrm{dd}}-x_{l}}\right)}{x_{\mathrm{ddd}}}\right)}{{\left(x_{\mathrm{dd}}-x_{l}\right)}^2}\right)}{T_{\mathrm{dd}}}$
      | Automatically generated on 2025-11-01 18:30:06 .
  State_E_fd_SG_D_1_d5aee : Inport
  State_psi_fd_SG_D_1_c7574 : Inport  Port=2
  State_psi_1d_SG_D_1_1742e : Inport  Port=3
  State_psi_fd_SG_D_1_fe3bf : Inport  Port=4
  State_psi_1d_SG_D_1_b3018 : Inport  Port=5
  State_psi_d_SG_D_1_a13b4 : Inport  Port=6
  State_psi_fd_SG_D_1_1eed0 : Inport  Port=7
  State_psi_1d_SG_D_1_10652 : Inport  Port=8
  State_psi_d_SG_D_1_482bf : Inport  Port=9
  State_psi_fd_SG_D_1_e31c3 : Inport  Port=10
  Add_1720d : Sum
  Add_bb906 : Sum
  Constant_-1_1333f : Constant  Value=-1
  Constant_-1_82476 : Constant  Value=-1
  Constant_-1_82d8b : Constant  Value=-1
  Constant_2.0_a0827 : Constant  Value=2.0
  Constant_T_dd_f9492 : Constant  Value=T_dd
  Constant_x_d_812da : Constant  Value=x_d
  Constant_x_dd_167be : Constant  Value=x_dd
  Constant_x_dd_26fe3 : Constant  Value=x_dd
  Constant_x_dd_2eed3 : Constant  Value=x_dd
  Constant_x_dd_3dcc5 : Constant  Value=x_dd
  Constant_x_dd_87f6b : Constant  Value=x_dd
  Constant_x_dd_881dc : Constant  Value=x_dd
  Constant_x_dd_997de : Constant  Value=x_dd
  Constant_x_dd_b7a6f : Constant  Value=x_dd
  Constant_x_dd_c5701 : Constant  Value=x_dd
  Constant_x_dd_cd806 : Constant  Value=x_dd
  Constant_x_ddd_1b009 : Constant  Value=x_ddd
  Constant_x_ddd_1ce56 : Constant  Value=x_ddd
  Constant_x_ddd_3d662 : Constant  Value=x_ddd
  Constant_x_ddd_69e6e : Constant  Value=x_ddd
  Constant_x_ddd_8d513 : Constant  Value=x_ddd
  Constant_x_ddd_d9397 : Constant  Value=x_ddd
  Constant_x_ddd_e6de9 : Constant  Value=x_ddd
  Constant_x_l_00866 : Constant  Value=x_l
  Constant_x_l_16e4e : Constant  Value=x_l
  Constant_x_l_4def4 : Constant  Value=x_l
  Constant_x_l_69cb2 : Constant  Value=x_l
  Constant_x_l_6ae05 : Constant  Value=x_l
  Constant_x_l_b178b : Constant  Value=x_l
  Constant_x_l_b3098 : Constant  Value=x_l
  Constant_x_l_cab71 : Constant  Value=x_l
  Divide_3ac01 : Product  Inputs=*/
  Divide_5673c : Product  Inputs=*/
  Divide_68a3b : Product  Inputs=*/
  Divide_74b6b : Product  Inputs=*/
  Divide_74d50 : Product  Inputs=*/
  Divide_9f3cf : Product  Inputs=*/
  Divide_c1b9a : Product  Inputs=*/
  Divide_dab06 : Product  Inputs=*/
  Power_65fa4 : Math  Operator=pow
  Product_2e75d : Product
  Product_7422e : Product
  Product_7d481 : Product
  Product_864e2 : Product
  Product_95af9 : Product
  Product_9f460 : Product
  Product_bfa26 : Product
  Product_ccb12 : Product
  Product_cd1fd : Product
  Product_de787 : Product
  Subtract_000a7 : Sum  Inputs=+-
  Subtract_05729 : Sum  Inputs=+-
  Subtract_061e5 : Sum  Inputs=+-
  Subtract_14d9c : Sum  Inputs=+-
  Subtract_1922f : Sum  Inputs=+-
  Subtract_1c261 : Sum  Inputs=+-
  Subtract_1d6c3 : Sum  Inputs=+-
  Subtract_1eb5b : Sum  Inputs=+-
  Subtract_34381 : Sum  Inputs=+-
  Subtract_47802 : Sum  Inputs=+-
  Subtract_5a8fc : Sum  Inputs=+-
  Subtract_63500 : Sum  Inputs=+-
  Subtract_68f7b : Sum  Inputs=+-
  Subtract_6d147 : Sum  Inputs=+-
  Subtract_6ee82 : Sum  Inputs=+-
  Subtract_bb2b5 : Sum  Inputs=+-
  Subtract_bb627 : Sum  Inputs=+-
  Subtract_c7510 : Sum  Inputs=+-
  Subtract_e6f06 : Sum  Inputs=+-
  Blockout_d_psi_fd_SG_D_1_f96ae : Outport
  wires:
  State_psi_d_SG_D_1_a13b4/1 -> Add_1720d/2
  Constant_x_dd_167be/1 -> Subtract_47802/1
  Product_2e75d/1 -> Divide_68a3b/1
  Subtract_34381/1 -> Product_2e75d/2
  Subtract_6ee82/1 -> Product_95af9/2
  Product_864e2/1 -> Product_2e75d/1
  Constant_x_dd_2eed3/1 -> Subtract_34381/1
  Constant_x_l_16e4e/1 -> Subtract_e6f06/2
  Constant_-1_82d8b/1 -> Product_864e2/1
  Subtract_e6f06/1 -> Product_95af9/1
  Constant_x_l_cab71/1 -> Subtract_47802/2
  Constant_x_ddd_e6de9/1 -> Subtract_34381/2
  State_psi_1d_SG_D_1_b3018/1 -> Product_864e2/2
  Constant_x_ddd_1ce56/1 -> Subtract_061e5/1
  Constant_x_l_4def4/1 -> Subtract_061e5/2
  State_E_fd_SG_D_1_d5aee/1 -> Subtract_1d6c3/1
  Divide_68a3b/1 -> Add_1720d/1
  Subtract_47802/1 -> Divide_68a3b/2
  State_psi_fd_SG_D_1_1eed0/1 -> Product_7422e/1
  Constant_x_ddd_69e6e/1 -> Divide_5673c/2
  Subtract_061e5/1 -> Product_7422e/2
  Constant_x_dd_997de/1 -> Subtract_1922f/1
  Constant_x_dd_b7a6f/1 -> Subtract_14d9c/1
  State_psi_fd_SG_D_1_c7574/1 -> Subtract_1d6c3/2
  Constant_x_l_69cb2/1 -> Subtract_1922f/2
  Product_7422e/1 -> Divide_9f3cf/1
  Constant_-1_1333f/1 -> Product_7d481/1
  Subtract_1922f/1 -> Divide_9f3cf/2
  Constant_x_dd_c5701/1 -> Subtract_e6f06/1
  Add_1720d/1 -> Subtract_6ee82/1
  Constant_x_l_b178b/1 -> Subtract_14d9c/2
  Divide_9f3cf/1 -> Subtract_6ee82/2
  Divide_74d50/1 -> Subtract_05729/1
  Constant_-1_82476/1 -> Product_9f460/1
  State_psi_1d_SG_D_1_10652/1 -> Product_9f460/2
  Constant_x_dd_26fe3/1 -> Subtract_c7510/1
  Subtract_1eb5b/1 -> Product_7d481/2
  Constant_x_ddd_1b009/1 -> Subtract_c7510/2
  Product_9f460/1 -> Product_bfa26/1
  Constant_2.0_a0827/1 -> Power_65fa4/2
  Product_bfa26/1 -> Divide_74b6b/1
  Subtract_05729/1 -> Product_ccb12/2
  Subtract_c7510/1 -> Product_bfa26/2
  State_psi_d_SG_D_1_482bf/1 -> Add_bb906/2
  Constant_x_dd_87f6b/1 -> Subtract_68f7b/1
  Constant_x_l_00866/1 -> Subtract_68f7b/2
  Constant_x_dd_3dcc5/1 -> Subtract_1eb5b/1
  Divide_5673c/1 -> Subtract_000a7/2
  Constant_x_ddd_3d662/1 -> Subtract_bb2b5/1
  Constant_x_ddd_d9397/1 -> Subtract_1eb5b/2
  Constant_x_l_6ae05/1 -> Subtract_bb2b5/2
  Subtract_bb2b5/1 -> Product_cd1fd/2
  State_psi_1d_SG_D_1_1742e/1 -> Subtract_63500/1
  Product_cd1fd/1 -> Divide_3ac01/1
  State_psi_fd_SG_D_1_fe3bf/1 -> Subtract_63500/2
  State_psi_fd_SG_D_1_e31c3/1 -> Product_cd1fd/1
  Product_95af9/1 -> Divide_5673c/1
  Divide_74b6b/1 -> Add_bb906/1
  Subtract_68f7b/1 -> Divide_74b6b/2
  Constant_x_dd_cd806/1 -> Subtract_6d147/1
  Constant_x_l_b3098/1 -> Subtract_6d147/2
  Divide_3ac01/1 -> Subtract_bb627/2
  Subtract_63500/1 -> Subtract_000a7/1
  Subtract_6d147/1 -> Divide_3ac01/2
  Subtract_000a7/1 -> Product_de787/2
  Product_7d481/1 -> Product_de787/1
  Subtract_14d9c/1 -> Power_65fa4/1
  Add_bb906/1 -> Subtract_bb627/1
  Product_de787/1 -> Divide_74d50/1
  Power_65fa4/1 -> Divide_74d50/2
  Subtract_bb627/1 -> Divide_dab06/1
  Constant_x_ddd_8d513/1 -> Divide_dab06/2
  Constant_x_d_812da/1 -> Subtract_5a8fc/1
  Constant_x_dd_881dc/1 -> Subtract_5a8fc/2
  Divide_dab06/1 -> Subtract_05729/2
  Subtract_5a8fc/1 -> Product_ccb12/1
  Subtract_1d6c3/1 -> Subtract_1c261/1
  Product_ccb12/1 -> Subtract_1c261/2
  Subtract_1c261/1 -> Divide_c1b9a/1
  Constant_T_dd_f9492/1 -> Divide_c1b9a/2
  Divide_c1b9a/1 -> Blockout_d_psi_fd_SG_D_1_f96ae/1

== system IEEE30_case/SG_D_1/d_psi_gq_SG_D_1_block ==
  note: d_psi_gq_SG_D_1 in IEEE30_case
      | $-\frac{\psi _{\mathrm{gq},\mathrm{SG},D,1}+\left(x_{q}-x_{\mathrm{qd}}\right)\,\left(\frac{\psi _{q,\mathrm{SG},D,1}+\frac{\psi _{\mathrm{gq},\mathrm{SG},D,1}\,\left(x_{l}-x_{\mathrm{qdd}}\right)}{x_{l}-x_{\mathrm{qd}}}+\frac{\psi _{\mathrm{kq},\mathrm{SG},D,1}\,\left(x_{\mathrm{qd}}-x_{\mathrm{qdd}}\right)}{x_{l}-x_{\mathrm{qd}}}}{x_{\mathrm{qdd}}}+\frac{\left(x_{\mathrm{qd}}-x_{\mathrm{qdd}}\right)\,\left(\psi _{\mathrm{gq},\mathrm{SG},D,1}+\psi _{\mathrm{kq},\mathrm{SG},D,1}+\frac{\left(x_{l}-x_{\mathrm{qd}}\right)\,\left(\psi _{q,\mathrm{SG},D,1}+\frac{\psi _{\mathrm{gq},\mathrm{SG},D,1}\,\left(x_{l}-x_{\mathrm{qdd}}\right)}{x_{l}-x_{\mathrm{qd}}}+\frac{\psi _{\mathrm{kq},\mathrm{SG},D,1}\,\left(x_{\mathrm{qd}}-x_{\mathrm{qdd}}\right)}{x_{l}-x_{\mathrm{qd}}}\right)}{x_{\mathrm{qdd}}}\right)}{{\left(x_{l}-x_{\mathrm{qd}}\right)}^2}\right)}{T_{\mathrm{qd}}}$
      | Automatically generated on 2025-11-01 18:30:14 .
  State_psi_gq_SG_D_1_332f7 : Inport
  State_psi_gq_SG_D_1_b0dac : Inport  Port=2
  State_psi_kq_SG_D_1_13d6b : Inport  Port=3
  State_psi_gq_SG_D_1_2cb53 : Inport  Port=4
  State_psi_kq_SG_D_1_4933d : Inport  Port=5
  State_psi_q_SG_D_1_31e6a : Inport  Port=6
  State_psi_gq_SG_D_1_3b2a6 : Inport  Port=7
  State_psi_kq_SG_D_1_372ae : Inport  Port=8
  State_psi_q_SG_D_1_64712 : Inport  Port=9
  Add_0bda5 : Sum
  Add_25ad5 : Sum
  Add_26367 : Sum
  Add_3a3ae : Sum
  Add_44f0d : Sum
  Add_88617 : Sum
  Add_ace86 : Sum
  Add_b2cb7 : Sum
  Add_b5122 : Sum
  Add_d8619 : Sum
  Add_e5e69 : Sum
  Add_f1b0b : Sum
  Constant_-1_02524 : Constant  Value=-1
  Constant_-1_2526b : Constant  Value=-1
  Constant_-1_{42169,75699,97200,97308} (4 alike) : Constant  Value=-1
  Constant_-1_5ebde : Constant  Value=-1
  Constant_-1_6bc2a : Constant  Value=-1
  Constant_-1_a12b2 : Constant  Value=-1
  Constant_-1_b7f1e : Constant  Value=-1
  Constant_2.0_e154a : Constant  Value=2.0
  Constant_T_qd_228ea : Constant  Value=T_qd
  Constant_x_l_1f290 : Constant  Value=x_l
  Constant_x_l_536d4 : Constant  Value=x_l
  Constant_x_l_58b27 : Constant  Value=x_l
  Constant_x_l_66bdc : Constant  Value=x_l
  Constant_x_l_6f6a2 : Constant  Value=x_l
  Constant_x_l_6f785 : Constant  Value=x_l
  Constant_x_l_70e3f : Constant  Value=x_l
  Constant_x_l_8fe40 : Constant  Value=x_l
  Constant_x_q_a4e50 : Constant  Value=x_q
  Constant_x_qd_2473f : Constant  Value=x_qd
  Constant_x_qd_2528b : Constant  Value=x_qd
  Constant_x_qd_43941 : Constant  Value=x_qd
  Constant_x_qd_8e3e6 : Constant  Value=x_qd
  Constant_x_qd_91883 : Constant  Value=x_qd
  Constant_x_qd_9e5a5 : Constant  Value=x_qd
  Constant_x_qd_acd23 : Constant  Value=x_qd
  Constant_x_qd_b0f27 : Constant  Value=x_qd
  Constant_x_qd_e370d : Constant  Value=x_qd
  Constant_x_qd_e747c : Constant  Value=x_qd
  Constant_x_qdd_3c027 : Constant  Value=x_qdd
  Constant_x_qdd_3eb02 : Constant  Value=x_qdd
  Constant_x_qdd_7a339 : Constant  Value=x_qdd
  Constant_x_qdd_83c03 : Constant  Value=x_qdd
  Constant_x_qdd_d7a4b : Constant  Value=x_qdd
  Constant_x_qdd_e155f : Constant  Value=x_qdd
  Constant_x_qdd_fe408 : Constant  Value=x_qdd
  Divide_11a05 : Product  Inputs=*/
  Divide_177f7 : Product  Inputs=*/
  Divide_3a79a : Product  Inputs=*/
  Divide_57fa5 : Product  Inputs=*/
  Divide_92f73 : Product  Inputs=*/
  Divide_be839 : Product  Inputs=*/
  Divide_da978 : Product  Inputs=*/
  Divide_fc537 : Product  Inputs=*/
  Power_e360c : Math  Operator=pow
  Product_09d3c : Product
  Product_09d42 : Product
  Product_0dcfe : Product
  Product_181b2 : Product
  Product_19d57 : Product
  Product_1c013 : Product
  Product_1c689 : Product
  Product_34dd6 : Product
  Product_3685a : Product
  Product_57ee3 : Product
  Product_aa4b3 : Product
  Product_af8f0 : Product
  Product_b3645 : Product
  Product_b8e34 : Product
  Product_bc783 : Product
  Product_d4808 : Product
  Product_f199b : Product
  Subtract_09c87 : Sum  Inputs=+-
  Subtract_496e5 : Sum  Inputs=+-
  Subtract_624bf : Sum  Inputs=+-
  Subtract_a962c : Sum  Inputs=+-
  Subtract_af226 : Sum  Inputs=+-
  Subtract_cba71 : Sum  Inputs=+-
  Subtract_e30bf : Sum  Inputs=+-
  Subtract_ecc0d : Sum  Inputs=+-
  Blockout_d_psi_gq_SG_D_1_8e30a : Outport
  wires:
  State_psi_gq_SG_D_1_2cb53/1 -> Product_d4808/1
  Constant_-1_75699/1 -> Product_57ee3/1
  Divide_fc537/1 -> Subtract_cba71/1
  Add_ace86/1 -> Divide_fc537/2
  Product_0dcfe/1 -> Add_b5122/1
  Constant_x_qd_8e3e6/1 -> Add_26367/2
  Constant_-1_6bc2a/1 -> Product_0dcfe/1
  Constant_x_qdd_7a339/1 -> Add_b5122/2
  Constant_x_l_66bdc/1 -> Product_57ee3/2
  Constant_x_l_8fe40/1 -> Product_0dcfe/2
  Constant_-1_a12b2/1 -> Product_1c689/1
  Constant_x_qd_b0f27/1 -> Subtract_624bf/1
  Constant_x_qdd_3eb02/1 -> Divide_92f73/2
  Constant_x_l_58b27/1 -> Product_1c689/2
  Constant_x_qdd_3c027/1 -> Subtract_624bf/2
  Subtract_cba71/1 -> Add_0bda5/1
  Add_b5122/1 -> Product_d4808/2
  Product_d4808/1 -> Divide_fc537/1
  Product_57ee3/1 -> Add_ace86/1
  Constant_x_qd_2528b/1 -> Add_ace86/2
  State_psi_kq_SG_D_1_4933d/1 -> Product_19d57/1
  Product_1c689/1 -> Add_3a3ae/1
  Subtract_624bf/1 -> Product_19d57/2
  Constant_x_qd_e370d/1 -> Add_3a3ae/2
  Product_19d57/1 -> Divide_11a05/1
  Add_3a3ae/1 -> Divide_11a05/2
  Constant_-1_97308/1 -> Product_1c013/1
  Constant_-1_5ebde/1 -> Product_aa4b3/1
  Add_f1b0b/1 -> Divide_177f7/2
  Product_3685a/1 -> Add_d8619/1
  Subtract_ecc0d/1 -> Product_bc783/2
  Constant_x_l_536d4/1 -> Product_aa4b3/2
  Divide_11a05/1 -> Subtract_cba71/2
  Subtract_af226/1 -> Product_b3645/1
  Constant_-1_02524/1 -> Product_f199b/1
  Constant_-1_2526b/1 -> Product_b8e34/1
  Constant_x_l_1f290/1 -> Product_f199b/2
  Constant_x_l_70e3f/1 -> Product_b8e34/2
  Constant_x_qd_43941/1 -> Add_f1b0b/2
  Product_aa4b3/1 -> Add_26367/1
  State_psi_q_SG_D_1_31e6a/1 -> Add_0bda5/2
  Product_b8e34/1 -> Add_e5e69/1
  Constant_x_qdd_d7a4b/1 -> Add_e5e69/2
  Constant_-1_b7f1e/1 -> Product_09d3c/1
  Constant_x_qd_91883/1 -> Add_d8619/2
  Add_26367/1 -> Product_34dd6/1
  Constant_x_l_6f6a2/1 -> Product_09d3c/2
  Constant_-1_42169/1 -> Product_3685a/1
  Constant_x_qd_2473f/1 -> Subtract_ecc0d/1
  Product_34dd6/1 -> Divide_92f73/1
  Constant_x_l_6f785/1 -> Product_3685a/2
  Divide_57fa5/1 -> Subtract_a962c/1
  Constant_x_qdd_e155f/1 -> Subtract_ecc0d/2
  Add_0bda5/1 -> Product_34dd6/2
  State_psi_gq_SG_D_1_3b2a6/1 -> Product_181b2/1
  Add_e5e69/1 -> Product_181b2/2
  Product_09d3c/1 -> Add_f1b0b/1
  State_psi_kq_SG_D_1_372ae/1 -> Product_bc783/1
  Add_d8619/1 -> Divide_be839/2
  State_psi_gq_SG_D_1_b0dac/1 -> Add_44f0d/1
  Constant_x_qd_acd23/1 -> Subtract_496e5/1
  Constant_x_qdd_fe408/1 -> Subtract_496e5/2
  Product_bc783/1 -> Divide_be839/1
  State_psi_kq_SG_D_1_13d6b/1 -> Add_44f0d/2
  Product_181b2/1 -> Divide_177f7/1
  Subtract_496e5/1 -> Product_1c013/2
  Add_44f0d/1 -> Subtract_09c87/1
  Divide_92f73/1 -> Subtract_09c87/2
  Product_f199b/1 -> Add_88617/1
  Constant_x_qd_e747c/1 -> Add_88617/2
  Divide_177f7/1 -> Subtract_e30bf/1
  Divide_be839/1 -> Subtract_e30bf/2
  Product_1c013/1 -> Product_09d42/1
  Subtract_09c87/1 -> Product_09d42/2
  Add_88617/1 -> Power_e360c/1
  Constant_2.0_e154a/1 -> Power_e360c/2
  Subtract_e30bf/1 -> Add_25ad5/1
  State_psi_q_SG_D_1_64712/1 -> Add_25ad5/2
  Product_09d42/1 -> Divide_57fa5/1
  Power_e360c/1 -> Divide_57fa5/2
  Add_25ad5/1 -> Divide_3a79a/1
  Constant_x_qdd_83c03/1 -> Divide_3a79a/2
  Constant_x_q_a4e50/1 -> Subtract_af226/1
  Constant_x_qd_9e5a5/1 -> Subtract_af226/2
  Divide_3a79a/1 -> Subtract_a962c/2
  Constant_-1_97200/1 -> Product_af8f0/1
  State_psi_gq_SG_D_1_332f7/1 -> Product_af8f0/2
  Subtract_a962c/1 -> Product_b3645/2
  Product_af8f0/1 -> Add_b2cb7/1
  Product_b3645/1 -> Add_b2cb7/2
  Add_b2cb7/1 -> Divide_da978/1
  Constant_T_qd_228ea/1 -> Divide_da978/2
  Divide_da978/1 -> Blockout_d_psi_gq_SG_D_1_8e30a/1
